simulink model "Copy_of_Scenario_MinimumExample_TwithoutTrafficLights"  (R2021a)
settings: Solver=VariableStepAuto  StartTime=0.0  StopTime=10.0  RelTol=1e-3
model workspace (MAT data in the model file):
  Kz_dif : Simulink.Parameter (value not decoded)
  Kz_il : Simulink.Parameter (value not decoded)
  Kz_ir : Simulink.Parameter (value not decoded)
  Kz_is : Simulink.Parameter (value not decoded)
  Kz_long : Simulink.Parameter (value not decoded)
  Kz_pre : Simulink.Parameter (value not decoded)
  L_dif : Simulink.Parameter (value not decoded)
  L_il : Simulink.Parameter (value not decoded)
  L_ir : Simulink.Parameter (value not decoded)
  L_is : Simulink.Parameter (value not decoded)
  L_long : Simulink.Parameter (value not decoded)
  L_pre : Simulink.Parameter (value not decoded)
  Lc : Simulink.Parameter (value not decoded)
  Rk : Simulink.Parameter (value not decoded)
  Tz_dif : Simulink.Parameter (value not decoded)
  Tz_il : Simulink.Parameter (value not decoded)
  Tz_ir : Simulink.Parameter (value not decoded)
  Tz_is : Simulink.Parameter (value not decoded)
  Tz_long : Simulink.Parameter (value not decoded)
  Tz_pre : Simulink.Parameter (value not decoded)
  ds : Simulink.Parameter (value not decoded)
  dt : Simulink.Parameter (value not decoded)
  v : Simulink.Parameter (value not decoded)
symbols that are objects in the model workspace (value not decoded): Kz_dif, Kz_il, Kz_ir, Kz_is, Kz_long, Kz_pre, Rk, Tz_dif, Tz_il, Tz_ir, Tz_is, Tz_long, Tz_pre
undefined symbols (not defined in the file): green_duration_l
libraries: StreetLanesLibrary x72, EdgesLibrary x58, SourcesAndSinksLibrary x12, simulink x12, LightsLibrary x2
(part 2 of 2)

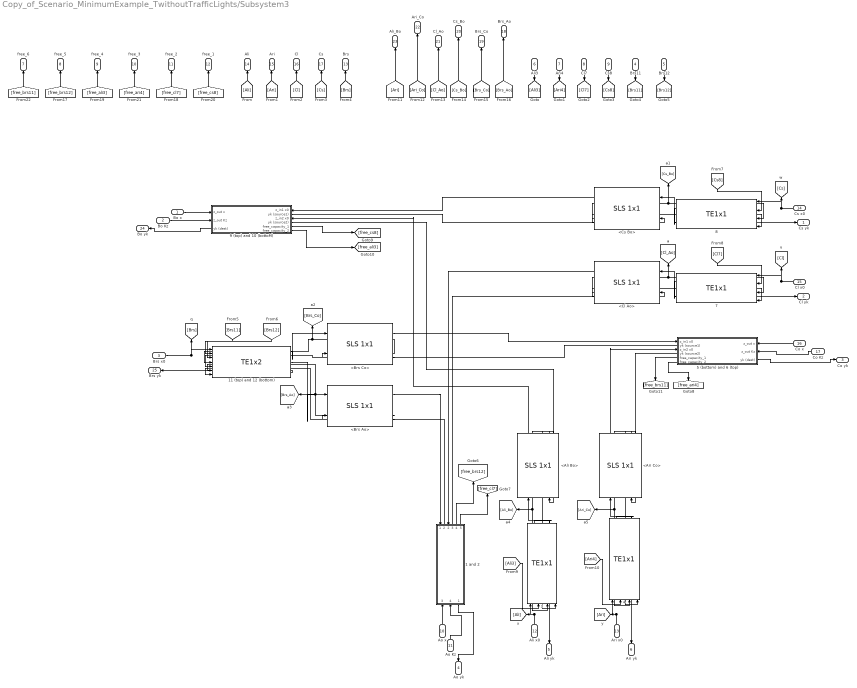
== system Copy_of_Scenario_MinimumExample_TwithoutTrafficLights/Subsystem3 ==
  Bo x : Inport
  Bo Kz : Inport  Port=2
  Brs x0 : Inport  Port=3
  Brs11 : Inport  Port=4
  Brs12 : Inport  Port=5
  Ali3 : Inport  Port=6
  Ari4 : Inport  Port=7
  Cl7 : Inport  Port=8
  Cs8 : Inport  Port=9
  Ao x : Inport  Port=10
  Ao Kz : Inport  Port=11
  Ali x0 : Inport  Port=12
  Ari x0 : Inport  Port=13
  Cs x0 : Inport  Port=14
  Cl x0 : Inport  Port=15
  Co x : Inport  Port=16
  Co Kz : Inport  Port=17
  1 and 2 : Subsystem  AncestorBlock=EdgesLibrary/SE2x1  mask{Rk1=Rk, Rk2=Rk}
      mask prompts: Rk1 "Rk (input 1)"; Rk2 "Rk (input 2)"
      settings: PortSchema="{\"entries\":[{\"content\":{\"sides\":[{\"content\":{\"connectorIds\":[\"In1\",\"Out2\",\"In2\",\"Out3\",\"Out4\",\"Out5\"]},\"type\":\"ConnectorPlacement.EquallySpacedRectSide\",\"uuid\":\"eb102e1f-8f68-4819-b192-9ed8ea7965cd\"},{\"content\":{\"connectorIds\":[\"In3\",\"In4\",\"Out1\"],\"side\":\"RIGHT\"},\"type\":\"ConnectorPlacement.EquallySpacedRectSide\",\"uuid\":\"0a8d41cc-2128-49e0-9ce9-20439c8bfca2\"},{\"content\":{\"connectorIds\":[],\"side\":\"TOP\"},\"type\":\"ConnectorPlacement.EquallySpacedRectSide\",\"uuid\":\"ce1e229b-7216-4f3c-b1ef-7720ca51f1c4\"}]},\"type\":\"ConnectorPlacement.EquallySpacedConnector\",\"uuid\":\"c8e8c67c-b38f-484f-95e7-011277152545\"}],\"packageUris\":[\"http://schema.mathworks.com/mf0/Connector/R2020b\"],\"version\":\"1.0\"}"
      mask Display:
      | image('$imagefile'); % Use "Edit Image" on toolstrip to change.
      | disp('Simple Edge 2x1\n\n\n');
      | Rk1 = get_param(gcb,'Rk1');
      | Rk2 = get_param(gcb, 'Rk2');
      | disp(['Rk1 = ', Rk1, ' | Rk2 =  ', Rk2])
  11 (top) and 12 (bottom) : EdgesLibrary/TE1x2  Rk1=0.5*Rk  Rk2=0.5*Rk
  {3..4,7..8} (4 alike) : EdgesLibrary/TE1x1  Rk=Rk
  5 (bottom) and 6 (top) : Subsystem  AncestorBlock=EdgesLibrary/SE2x1  mask{Rk1=Rk, Rk2=Rk}
      mask prompts: Rk1 "Rk (input 1)"; Rk2 "Rk (input 2)"
      settings: PortSchema="{\"entries\":[{\"content\":{\"sides\":[{\"content\":{\"connectorIds\":[\"In1\",\"Out2\",\"In2\",\"Out3\",\"Out4\",\"Out5\"]},\"type\":\"ConnectorPlacement.EquallySpacedRectSide\",\"uuid\":\"eb102e1f-8f68-4819-b192-9ed8ea7965cd\"},{\"content\":{\"connectorIds\":[\"In3\",\"In4\",\"Out1\"],\"side\":\"RIGHT\"},\"type\":\"ConnectorPlacement.EquallySpacedRectSide\",\"uuid\":\"0a8d41cc-2128-49e0-9ce9-20439c8bfca2\"},{\"content\":{\"connectorIds\":[],\"side\":\"TOP\"},\"type\":\"ConnectorPlacement.EquallySpacedRectSide\",\"uuid\":\"ce1e229b-7216-4f3c-b1ef-7720ca51f1c4\"}]},\"type\":\"ConnectorPlacement.EquallySpacedConnector\",\"uuid\":\"c8e8c67c-b38f-484f-95e7-011277152545\"}],\"packageUris\":[\"http://schema.mathworks.com/mf0/Connector/R2020b\"],\"version\":\"1.0\"}"
      mask Display:
      | image('$imagefile'); % Use "Edit Image" on toolstrip to change.
      | disp('Simple Edge 2x1\n\n\n');
      | Rk1 = get_param(gcb,'Rk1');
      | Rk2 = get_param(gcb, 'Rk2');
      | disp(['Rk1 = ', Rk1, ' | Rk2 =  ', Rk2])
  9 (top) and 10 (bottoM) : Subsystem  AncestorBlock=EdgesLibrary/SE2x1  mask{Rk1=Rk, Rk2=Rk}
      mask prompts: Rk1 "Rk (input 1)"; Rk2 "Rk (input 2)"
      settings: PortSchema="{\"entries\":[{\"content\":{\"sides\":[{\"content\":{\"connectorIds\":[\"In1\",\"Out2\",\"In2\",\"Out3\",\"Out4\",\"Out5\"]},\"type\":\"ConnectorPlacement.EquallySpacedRectSide\",\"uuid\":\"eb102e1f-8f68-4819-b192-9ed8ea7965cd\"},{\"content\":{\"connectorIds\":[\"In3\",\"In4\",\"Out1\"],\"side\":\"RIGHT\"},\"type\":\"ConnectorPlacement.EquallySpacedRectSide\",\"uuid\":\"0a8d41cc-2128-49e0-9ce9-20439c8bfca2\"},{\"content\":{\"connectorIds\":[],\"side\":\"TOP\"},\"type\":\"ConnectorPlacement.EquallySpacedRectSide\",\"uuid\":\"ce1e229b-7216-4f3c-b1ef-7720ca51f1c4\"}]},\"type\":\"ConnectorPlacement.EquallySpacedConnector\",\"uuid\":\"c8e8c67c-b38f-484f-95e7-011277152545\"}],\"packageUris\":[\"http://schema.mathworks.com/mf0/Connector/R2020b\"],\"version\":\"1.0\"}"
      mask Display:
      | image('$imagefile'); % Use "Edit Image" on toolstrip to change.
      | disp('Simple Edge 2x1\n\n\n');
      | Rk1 = get_param(gcb,'Rk1');
      | Rk2 = get_param(gcb, 'Rk2');
      | disp(['Rk1 = ', Rk1, ' | Rk2 =  ', Rk2])
  <Ali Bo> : StreetLanesLibrary/SLS 1x1  Kz=Kz_left  Tz=Tz_left
  <Ari Co> : StreetLanesLibrary/SLS 1x1  Kz=Kz_right  Tz=Tz_right
  <Brs Ao> : StreetLanesLibrary/SLS 1x1  Kz=Kz_right  Tz=Tz_right
  <Brs Co> : StreetLanesLibrary/SLS 1x1  Kz=Kz_straight  Tz=Tz_straight
  <Cl Ao> : StreetLanesLibrary/SLS 1x1  Kz=Kz_left  Tz=Tz_left
  <Cs Bo> : StreetLanesLibrary/SLS 1x1  Kz=Kz_straight  Tz=Tz_straight
  Cs yk : Outport
  Cl yk : Outport  Port=2
  Co yk : Outport  Port=3
  Ao yk : Outport  Port=4
  Ali yk : Outport  Port=5
  Ari yk : Outport  Port=6
  free_6 : Outport  Port=7
  free_5 : Outport  Port=8
  free_4 : Outport  Port=9
  free_3 : Outport  Port=10
  free_2 : Outport  Port=11
  free_1 : Outport  Port=12
  Brs : Outport  Port=13
  Ali : Outport  Port=14
  Ari : Outport  Port=15
  Cl : Outport  Port=16
  Cs : Outport  Port=17
  Brs_Ao : Outport  Port=18
  Brs_Co : Outport  Port=19
  Cs_Bo : Outport  Port=20
  Cl_Ao : Outport  Port=21
  Ari_Co : Outport  Port=22
  Ali_Bo : Outport  Port=23
  Bo yk : Outport  Port=24
  Brs yk : Outport  Port=25
  wires:
  11 (top) and 12 (bottom)/2 -> <Brs Ao>/1
  11 (top) and 12 (bottom)/3 -> Brs yk/1
  3/2 -> Ali yk/1
  3/1 -> <Ali Bo>/1
  Ari x0/1 -> [Ari], 4/1
  <Cs Bo>/2 -> 9 (top) and 10 (bottoM)/1(z_in1 x0)
  <Cs Bo>/8 -> 8/4
  <Cl Ao>/8 -> 7/4
  Co x/1 -> 5 (bottom) and 6 (top)/3(z_out x)
  5 (bottom) and 6 (top)/1(yk (dest)) -> Co yk/1
  5 (bottom) and 6 (top)/3(yk (source2)) -> <Ari Co>/2
  <Ari Co>/8 -> 4/4
  <Ali Bo>/8 -> 3/4
  Ao x/1 -> 1 and 2/3(z_out x)
  Brs x0/1 -> 11 (top) and 12 (bottom)/1, [Brs]
  <Brs Co>/2 -> 5 (bottom) and 6 (top)/1(z_in1 x0)
  <Cl Ao>/7 -> [Cl_Ao], 7/3
  <Cl Ao>/2 -> 1 and 2/2(z_in2 x0)
  9 (top) and 10 (bottoM)/2(yk (source1)) -> <Cs Bo>/2
  <Ari Co>/2 -> 5 (bottom) and 6 (top)/2(z_in2 x0)
  7/1 -> <Cl Ao>/1
  Cl x0/1 -> [Cl], 7/1
  4/1 -> <Ari Co>/1
  <Ari Co>/7 -> 4/3, [Ari_Co]
  <Brs Ao>/2 -> 1 and 2/1(z_in1 x0)
  Ao Kz/1 -> 1 and 2/4(z_out Kz)
  <Brs Ao>/7 -> [Brs_Ao], 11 (top) and 12 (bottom)/6
  <Brs Ao>/8 -> 11 (top) and 12 (bottom)/7
  Co Kz/1 -> 5 (bottom) and 6 (top)/4(z_out Kz)
  8/2 -> Cs yk/1
  Bo Kz/1 -> 9 (top) and 10 (bottoM)/4(z_out Kz)
  1 and 2/3(yk (source2)) -> <Cl Ao>/2
  <Brs Co>/8 -> 11 (top) and 12 (bottom)/5
  [Brs12] -> 11 (top) and 12 (bottom)/3
  9 (top) and 10 (bottoM)/3(yk (source2)) -> <Ali Bo>/2
  <Ali Bo>/7 -> 3/3, [Ali_Bo]
  1 and 2/2(yk (source1)) -> <Brs Ao>/2
  Ali x0/1 -> [Ali], 3/1
  <Brs Co>/7 -> 11 (top) and 12 (bottom)/4, [Brs_Co]
  1 and 2/1(yk (dest)) -> Ao yk/1
  <Ali Bo>/2 -> 9 (top) and 10 (bottoM)/2(z_in2 x0)
  [Ari4] -> 4/2
  5 (bottom) and 6 (top)/2(yk (source1)) -> <Brs Co>/2
  8/1 -> <Cs Bo>/1
  4/2 -> Ari yk/1
  <Cs Bo>/7 -> 8/3, [Cs_Bo]
  Cs x0/1 -> [Cs], 8/1
  [Ali3] -> 3/2
  [Brs11] -> 11 (top) and 12 (bottom)/2
  11 (top) and 12 (bottom)/1 -> <Brs Co>/1
  Bo x/1 -> 9 (top) and 10 (bottoM)/3(z_out x)
  [Cl7] -> 7/2
  9 (top) and 10 (bottoM)/1(yk (dest)) -> Bo yk/1
  7/2 -> Cl yk/1
  [Cs8] -> 8/2
  [Ari] -> Ali_Bo/1
  [Ari_Co] -> Ari_Co/1
  [Cl_Ao] -> Cl_Ao/1
  [Cs_Bo] -> Cs_Bo/1
  [Brs_Co] -> Brs_Co/1
  [Brs_Ao] -> Brs_Ao/1
  [Ali] -> Ali/1
  [Ari] -> Ari/1
  [Cl] -> Cl/1
  [Cs] -> Cs/1
  [Brs] -> Brs/1
  Ali3/1 -> [Ali3]
  Ari4/1 -> [Ari4]
  Cl7/1 -> [Cl7]
  Cs8/1 -> [Cs8]
  Brs11/1 -> [Brs11]
  Brs12/1 -> [Brs12]
  1 and 2/4(free_capacity_1) -> [free_brs12]
  1 and 2/5(free_capacity_2) -> [free_cl7]
  9 (top) and 10 (bottoM)/4(free_capacity_1) -> [free_cs8]
  9 (top) and 10 (bottoM)/5(free_capacity_2) -> [free_ali3]
  5 (bottom) and 6 (top)/5(free_capacity_2) -> [free_ari4]
  5 (bottom) and 6 (top)/4(free_capacity_1) -> [free_brs11]
  [free_cs8] -> free_1/1
  [free_cl7] -> free_2/1
  [free_ari4] -> free_3/1
  [free_ali3] -> free_4/1
  [free_brs12] -> free_5/1
  [free_brs11] -> free_6/1

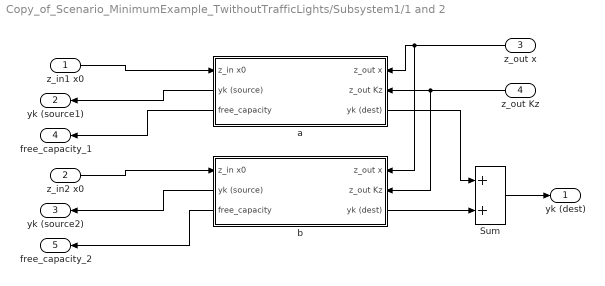
== system Copy_of_Scenario_MinimumExample_TwithoutTrafficLights/Subsystem1/1 and 2 ==
  z_in1 x0 : Inport
  z_in2 x0 : Inport  Port=2
  z_out x : Inport  Port=3
  z_out Kz : Inport  Port=4
  Sum : Sum
  a : Subsystem  AncestorBlock=EdgesLibrary/SE1x1  mask{Rk=Rk1}
      mask prompts: Rk "Rk (fixed flowrate, used when the flow is enabled)"
      mask help: This block serves to establish a flow between two Street Lane Segments. To archieve this, it connects one source-cell [z_in] to one destination-cell [z_out], and prompts a flow of cars with the rate Rk (Parameter) if and only if there are still cars at the end of [z_out] avaiable and if the capacity of [z_out] is not yet surpassed, i.e. (z_in x0 > 0 AND z_out Kz > z_out x), otherwise the flow is reduced to 0.
      settings: PortSchema="{\"entries\":[{\"content\":{\"sides\":[{\"content\":{\"connectorIds\":[\"In1\",\"Out2\",\"Out3\"]},\"type\":\"ConnectorPlacement.EquallySpacedRectSide\",\"uuid\":\"f9c1cf46-46ac-4011-8499-7a2e74fc4a3a\"},{\"content\":{\"connectorIds\":[\"In2\",\"In3\",\"Out1\"],\"side\":\"RIGHT\"},\"type\":\"ConnectorPlacement.EquallySpacedRectSide\",\"uuid\":\"f685a77a-a8b9-4a29-8679-dc3cbf3c2b7f\"},{\"content\":{\"connectorIds\":[],\"side\":\"TOP\"},\"type\":\"ConnectorPlacement.EquallySpacedRectSide\",\"uuid\":\"af8d715a-ddb3-4f5e-8163-596be4e65ef7\"}]},\"type\":\"ConnectorPlacement.EquallySpacedConnector\",\"uuid\":\"ace495d2-b7cd-4153-a555-4989f077c969\"}],\"packageUris\":[\"http://schema.mathworks.com/mf0/Connector/R2020b\"],\"version\":\"1.0\"}"
      mask Display:
      | image('$imagefile'); % Use "Edit Image" on toolstrip to change.
      | % image('$imagefile');
      | disp('Simple Edge 1x1 \n\n');
      | disp(['Rk = ', get_param(gcb,'Rk')])
  b : Subsystem  AncestorBlock=EdgesLibrary/SE1x1  mask{Rk=Rk2}
      mask prompts: Rk "Rk (fixed flowrate, used when the flow is enabled)"
      mask help: This block serves to establish a flow between two Street Lane Segments. To archieve this, it connects one source-cell [z_in] to one destination-cell [z_out], and prompts a flow of cars with the rate Rk (Parameter) if and only if there are still cars at the end of [z_out] avaiable and if the capacity of [z_out] is not yet surpassed, i.e. (z_in x0 > 0 AND z_out Kz > z_out x), otherwise the flow is reduced to 0.
      settings: PortSchema="{\"entries\":[{\"content\":{\"sides\":[{\"content\":{\"connectorIds\":[\"In1\",\"Out2\",\"Out3\"]},\"type\":\"ConnectorPlacement.EquallySpacedRectSide\",\"uuid\":\"f9c1cf46-46ac-4011-8499-7a2e74fc4a3a\"},{\"content\":{\"connectorIds\":[\"In2\",\"In3\",\"Out1\"],\"side\":\"RIGHT\"},\"type\":\"ConnectorPlacement.EquallySpacedRectSide\",\"uuid\":\"f685a77a-a8b9-4a29-8679-dc3cbf3c2b7f\"},{\"content\":{\"connectorIds\":[],\"side\":\"TOP\"},\"type\":\"ConnectorPlacement.EquallySpacedRectSide\",\"uuid\":\"af8d715a-ddb3-4f5e-8163-596be4e65ef7\"}]},\"type\":\"ConnectorPlacement.EquallySpacedConnector\",\"uuid\":\"ace495d2-b7cd-4153-a555-4989f077c969\"}],\"packageUris\":[\"http://schema.mathworks.com/mf0/Connector/R2020b\"],\"version\":\"1.0\"}"
      mask Display:
      | image('$imagefile'); % Use "Edit Image" on toolstrip to change.
      | % image('$imagefile');
      | disp('Simple Edge 1x1 \n\n');
      | disp(['Rk = ', get_param(gcb,'Rk')])
  yk (dest) : Outport
  yk (source1) : Outport  Port=2
  yk (source2) : Outport  Port=3
  free_capacity_1 : Outport  Port=4
  free_capacity_2 : Outport  Port=5
  wires:
  z_out Kz/1 -> b/3(z_out Kz), a/3(z_out Kz)
  Sum/1 -> yk (dest)/1
  z_out x/1 -> b/2(z_out x), a/2(z_out x)
  b/1(yk (dest)) -> Sum/2
  z_in1 x0/1 -> a/1(z_in x0)
  a/1(yk (dest)) -> Sum/1
  z_in2 x0/1 -> b/1(z_in x0)
  b/2(yk (source)) -> yk (source2)/1
  a/2(yk (source)) -> yk (source1)/1
  a/3(free_capacity) -> free_capacity_1/1
  b/3(free_capacity) -> free_capacity_2/1

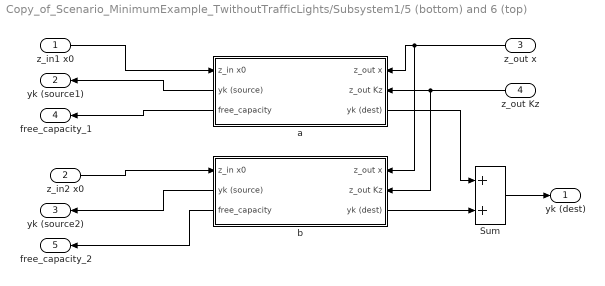
== system Copy_of_Scenario_MinimumExample_TwithoutTrafficLights/Subsystem1/5 (bottom) and 6 (top) ==
  z_in1 x0 : Inport
  z_in2 x0 : Inport  Port=2
  z_out x : Inport  Port=3
  z_out Kz : Inport  Port=4
  Sum : Sum
  a : Subsystem  AncestorBlock=EdgesLibrary/SE1x1  mask{Rk=Rk1}
      mask prompts: Rk "Rk (fixed flowrate, used when the flow is enabled)"
      mask help: This block serves to establish a flow between two Street Lane Segments. To archieve this, it connects one source-cell [z_in] to one destination-cell [z_out], and prompts a flow of cars with the rate Rk (Parameter) if and only if there are still cars at the end of [z_out] avaiable and if the capacity of [z_out] is not yet surpassed, i.e. (z_in x0 > 0 AND z_out Kz > z_out x), otherwise the flow is reduced to 0.
      settings: PortSchema="{\"entries\":[{\"content\":{\"sides\":[{\"content\":{\"connectorIds\":[\"In1\",\"Out2\",\"Out3\"]},\"type\":\"ConnectorPlacement.EquallySpacedRectSide\",\"uuid\":\"f9c1cf46-46ac-4011-8499-7a2e74fc4a3a\"},{\"content\":{\"connectorIds\":[\"In2\",\"In3\",\"Out1\"],\"side\":\"RIGHT\"},\"type\":\"ConnectorPlacement.EquallySpacedRectSide\",\"uuid\":\"f685a77a-a8b9-4a29-8679-dc3cbf3c2b7f\"},{\"content\":{\"connectorIds\":[],\"side\":\"TOP\"},\"type\":\"ConnectorPlacement.EquallySpacedRectSide\",\"uuid\":\"af8d715a-ddb3-4f5e-8163-596be4e65ef7\"}]},\"type\":\"ConnectorPlacement.EquallySpacedConnector\",\"uuid\":\"ace495d2-b7cd-4153-a555-4989f077c969\"}],\"packageUris\":[\"http://schema.mathworks.com/mf0/Connector/R2020b\"],\"version\":\"1.0\"}"
      mask Display:
      | image('$imagefile'); % Use "Edit Image" on toolstrip to change.
      | % image('$imagefile');
      | disp('Simple Edge 1x1 \n\n');
      | disp(['Rk = ', get_param(gcb,'Rk')])
  b : Subsystem  AncestorBlock=EdgesLibrary/SE1x1  mask{Rk=Rk2}
      mask prompts: Rk "Rk (fixed flowrate, used when the flow is enabled)"
      mask help: This block serves to establish a flow between two Street Lane Segments. To archieve this, it connects one source-cell [z_in] to one destination-cell [z_out], and prompts a flow of cars with the rate Rk (Parameter) if and only if there are still cars at the end of [z_out] avaiable and if the capacity of [z_out] is not yet surpassed, i.e. (z_in x0 > 0 AND z_out Kz > z_out x), otherwise the flow is reduced to 0.
      settings: PortSchema="{\"entries\":[{\"content\":{\"sides\":[{\"content\":{\"connectorIds\":[\"In1\",\"Out2\",\"Out3\"]},\"type\":\"ConnectorPlacement.EquallySpacedRectSide\",\"uuid\":\"f9c1cf46-46ac-4011-8499-7a2e74fc4a3a\"},{\"content\":{\"connectorIds\":[\"In2\",\"In3\",\"Out1\"],\"side\":\"RIGHT\"},\"type\":\"ConnectorPlacement.EquallySpacedRectSide\",\"uuid\":\"f685a77a-a8b9-4a29-8679-dc3cbf3c2b7f\"},{\"content\":{\"connectorIds\":[],\"side\":\"TOP\"},\"type\":\"ConnectorPlacement.EquallySpacedRectSide\",\"uuid\":\"af8d715a-ddb3-4f5e-8163-596be4e65ef7\"}]},\"type\":\"ConnectorPlacement.EquallySpacedConnector\",\"uuid\":\"ace495d2-b7cd-4153-a555-4989f077c969\"}],\"packageUris\":[\"http://schema.mathworks.com/mf0/Connector/R2020b\"],\"version\":\"1.0\"}"
      mask Display:
      | image('$imagefile'); % Use "Edit Image" on toolstrip to change.
      | % image('$imagefile');
      | disp('Simple Edge 1x1 \n\n');
      | disp(['Rk = ', get_param(gcb,'Rk')])
  yk (dest) : Outport
  yk (source1) : Outport  Port=2
  yk (source2) : Outport  Port=3
  free_capacity_1 : Outport  Port=4
  free_capacity_2 : Outport  Port=5
  wires:
  z_out Kz/1 -> b/3(z_out Kz), a/3(z_out Kz)
  Sum/1 -> yk (dest)/1
  z_out x/1 -> b/2(z_out x), a/2(z_out x)
  b/1(yk (dest)) -> Sum/2
  z_in1 x0/1 -> a/1(z_in x0)
  a/1(yk (dest)) -> Sum/1
  z_in2 x0/1 -> b/1(z_in x0)
  b/2(yk (source)) -> yk (source2)/1
  a/2(yk (source)) -> yk (source1)/1
  a/3(free_capacity) -> free_capacity_1/1
  b/3(free_capacity) -> free_capacity_2/1

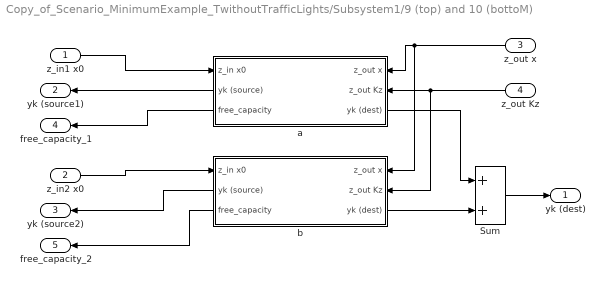
== system Copy_of_Scenario_MinimumExample_TwithoutTrafficLights/Subsystem1/9 (top) and 10 (bottoM) ==
  z_in1 x0 : Inport
  z_in2 x0 : Inport  Port=2
  z_out x : Inport  Port=3
  z_out Kz : Inport  Port=4
  Sum : Sum
  a : Subsystem  AncestorBlock=EdgesLibrary/SE1x1  mask{Rk=Rk1}
      mask prompts: Rk "Rk (fixed flowrate, used when the flow is enabled)"
      mask help: This block serves to establish a flow between two Street Lane Segments. To archieve this, it connects one source-cell [z_in] to one destination-cell [z_out], and prompts a flow of cars with the rate Rk (Parameter) if and only if there are still cars at the end of [z_out] avaiable and if the capacity of [z_out] is not yet surpassed, i.e. (z_in x0 > 0 AND z_out Kz > z_out x), otherwise the flow is reduced to 0.
      settings: PortSchema="{\"entries\":[{\"content\":{\"sides\":[{\"content\":{\"connectorIds\":[\"In1\",\"Out2\",\"Out3\"]},\"type\":\"ConnectorPlacement.EquallySpacedRectSide\",\"uuid\":\"f9c1cf46-46ac-4011-8499-7a2e74fc4a3a\"},{\"content\":{\"connectorIds\":[\"In2\",\"In3\",\"Out1\"],\"side\":\"RIGHT\"},\"type\":\"ConnectorPlacement.EquallySpacedRectSide\",\"uuid\":\"f685a77a-a8b9-4a29-8679-dc3cbf3c2b7f\"},{\"content\":{\"connectorIds\":[],\"side\":\"TOP\"},\"type\":\"ConnectorPlacement.EquallySpacedRectSide\",\"uuid\":\"af8d715a-ddb3-4f5e-8163-596be4e65ef7\"}]},\"type\":\"ConnectorPlacement.EquallySpacedConnector\",\"uuid\":\"ace495d2-b7cd-4153-a555-4989f077c969\"}],\"packageUris\":[\"http://schema.mathworks.com/mf0/Connector/R2020b\"],\"version\":\"1.0\"}"
      mask Display:
      | image('$imagefile'); % Use "Edit Image" on toolstrip to change.
      | % image('$imagefile');
      | disp('Simple Edge 1x1 \n\n');
      | disp(['Rk = ', get_param(gcb,'Rk')])
  b : Subsystem  AncestorBlock=EdgesLibrary/SE1x1  mask{Rk=Rk2}
      mask prompts: Rk "Rk (fixed flowrate, used when the flow is enabled)"
      mask help: This block serves to establish a flow between two Street Lane Segments. To archieve this, it connects one source-cell [z_in] to one destination-cell [z_out], and prompts a flow of cars with the rate Rk (Parameter) if and only if there are still cars at the end of [z_out] avaiable and if the capacity of [z_out] is not yet surpassed, i.e. (z_in x0 > 0 AND z_out Kz > z_out x), otherwise the flow is reduced to 0.
      settings: PortSchema="{\"entries\":[{\"content\":{\"sides\":[{\"content\":{\"connectorIds\":[\"In1\",\"Out2\",\"Out3\"]},\"type\":\"ConnectorPlacement.EquallySpacedRectSide\",\"uuid\":\"f9c1cf46-46ac-4011-8499-7a2e74fc4a3a\"},{\"content\":{\"connectorIds\":[\"In2\",\"In3\",\"Out1\"],\"side\":\"RIGHT\"},\"type\":\"ConnectorPlacement.EquallySpacedRectSide\",\"uuid\":\"f685a77a-a8b9-4a29-8679-dc3cbf3c2b7f\"},{\"content\":{\"connectorIds\":[],\"side\":\"TOP\"},\"type\":\"ConnectorPlacement.EquallySpacedRectSide\",\"uuid\":\"af8d715a-ddb3-4f5e-8163-596be4e65ef7\"}]},\"type\":\"ConnectorPlacement.EquallySpacedConnector\",\"uuid\":\"ace495d2-b7cd-4153-a555-4989f077c969\"}],\"packageUris\":[\"http://schema.mathworks.com/mf0/Connector/R2020b\"],\"version\":\"1.0\"}"
      mask Display:
      | image('$imagefile'); % Use "Edit Image" on toolstrip to change.
      | % image('$imagefile');
      | disp('Simple Edge 1x1 \n\n');
      | disp(['Rk = ', get_param(gcb,'Rk')])
  yk (dest) : Outport
  yk (source1) : Outport  Port=2
  yk (source2) : Outport  Port=3
  free_capacity_1 : Outport  Port=4
  free_capacity_2 : Outport  Port=5
  wires:
  z_out Kz/1 -> b/3(z_out Kz), a/3(z_out Kz)
  Sum/1 -> yk (dest)/1
  z_out x/1 -> b/2(z_out x), a/2(z_out x)
  b/1(yk (dest)) -> Sum/2
  z_in1 x0/1 -> a/1(z_in x0)
  a/1(yk (dest)) -> Sum/1
  z_in2 x0/1 -> b/1(z_in x0)
  b/2(yk (source)) -> yk (source2)/1
  a/2(yk (source)) -> yk (source1)/1
  a/3(free_capacity) -> free_capacity_1/1
  b/3(free_capacity) -> free_capacity_2/1

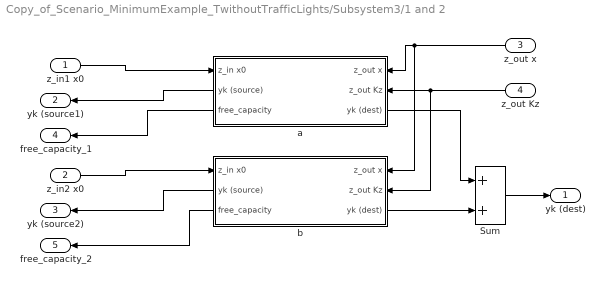
== system Copy_of_Scenario_MinimumExample_TwithoutTrafficLights/Subsystem3/1 and 2 ==
  z_in1 x0 : Inport
  z_in2 x0 : Inport  Port=2
  z_out x : Inport  Port=3
  z_out Kz : Inport  Port=4
  Sum : Sum
  a : Subsystem  AncestorBlock=EdgesLibrary/SE1x1  mask{Rk=Rk1}
      mask prompts: Rk "Rk (fixed flowrate, used when the flow is enabled)"
      mask help: This block serves to establish a flow between two Street Lane Segments. To archieve this, it connects one source-cell [z_in] to one destination-cell [z_out], and prompts a flow of cars with the rate Rk (Parameter) if and only if there are still cars at the end of [z_out] avaiable and if the capacity of [z_out] is not yet surpassed, i.e. (z_in x0 > 0 AND z_out Kz > z_out x), otherwise the flow is reduced to 0.
      settings: PortSchema="{\"entries\":[{\"content\":{\"sides\":[{\"content\":{\"connectorIds\":[\"In1\",\"Out2\",\"Out3\"]},\"type\":\"ConnectorPlacement.EquallySpacedRectSide\",\"uuid\":\"f9c1cf46-46ac-4011-8499-7a2e74fc4a3a\"},{\"content\":{\"connectorIds\":[\"In2\",\"In3\",\"Out1\"],\"side\":\"RIGHT\"},\"type\":\"ConnectorPlacement.EquallySpacedRectSide\",\"uuid\":\"f685a77a-a8b9-4a29-8679-dc3cbf3c2b7f\"},{\"content\":{\"connectorIds\":[],\"side\":\"TOP\"},\"type\":\"ConnectorPlacement.EquallySpacedRectSide\",\"uuid\":\"af8d715a-ddb3-4f5e-8163-596be4e65ef7\"}]},\"type\":\"ConnectorPlacement.EquallySpacedConnector\",\"uuid\":\"ace495d2-b7cd-4153-a555-4989f077c969\"}],\"packageUris\":[\"http://schema.mathworks.com/mf0/Connector/R2020b\"],\"version\":\"1.0\"}"
      mask Display:
      | image('$imagefile'); % Use "Edit Image" on toolstrip to change.
      | % image('$imagefile');
      | disp('Simple Edge 1x1 \n\n');
      | disp(['Rk = ', get_param(gcb,'Rk')])
  b : Subsystem  AncestorBlock=EdgesLibrary/SE1x1  mask{Rk=Rk2}
      mask prompts: Rk "Rk (fixed flowrate, used when the flow is enabled)"
      mask help: This block serves to establish a flow between two Street Lane Segments. To archieve this, it connects one source-cell [z_in] to one destination-cell [z_out], and prompts a flow of cars with the rate Rk (Parameter) if and only if there are still cars at the end of [z_out] avaiable and if the capacity of [z_out] is not yet surpassed, i.e. (z_in x0 > 0 AND z_out Kz > z_out x), otherwise the flow is reduced to 0.
      settings: PortSchema="{\"entries\":[{\"content\":{\"sides\":[{\"content\":{\"connectorIds\":[\"In1\",\"Out2\",\"Out3\"]},\"type\":\"ConnectorPlacement.EquallySpacedRectSide\",\"uuid\":\"f9c1cf46-46ac-4011-8499-7a2e74fc4a3a\"},{\"content\":{\"connectorIds\":[\"In2\",\"In3\",\"Out1\"],\"side\":\"RIGHT\"},\"type\":\"ConnectorPlacement.EquallySpacedRectSide\",\"uuid\":\"f685a77a-a8b9-4a29-8679-dc3cbf3c2b7f\"},{\"content\":{\"connectorIds\":[],\"side\":\"TOP\"},\"type\":\"ConnectorPlacement.EquallySpacedRectSide\",\"uuid\":\"af8d715a-ddb3-4f5e-8163-596be4e65ef7\"}]},\"type\":\"ConnectorPlacement.EquallySpacedConnector\",\"uuid\":\"ace495d2-b7cd-4153-a555-4989f077c969\"}],\"packageUris\":[\"http://schema.mathworks.com/mf0/Connector/R2020b\"],\"version\":\"1.0\"}"
      mask Display:
      | image('$imagefile'); % Use "Edit Image" on toolstrip to change.
      | % image('$imagefile');
      | disp('Simple Edge 1x1 \n\n');
      | disp(['Rk = ', get_param(gcb,'Rk')])
  yk (dest) : Outport
  yk (source1) : Outport  Port=2
  yk (source2) : Outport  Port=3
  free_capacity_1 : Outport  Port=4
  free_capacity_2 : Outport  Port=5
  wires:
  z_out Kz/1 -> b/3(z_out Kz), a/3(z_out Kz)
  Sum/1 -> yk (dest)/1
  z_out x/1 -> b/2(z_out x), a/2(z_out x)
  b/1(yk (dest)) -> Sum/2
  z_in1 x0/1 -> a/1(z_in x0)
  a/1(yk (dest)) -> Sum/1
  z_in2 x0/1 -> b/1(z_in x0)
  b/2(yk (source)) -> yk (source2)/1
  a/2(yk (source)) -> yk (source1)/1
  a/3(free_capacity) -> free_capacity_1/1
  b/3(free_capacity) -> free_capacity_2/1

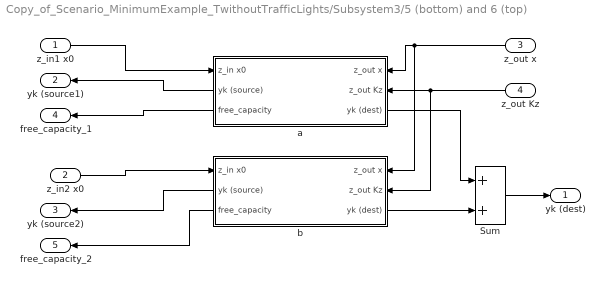
== system Copy_of_Scenario_MinimumExample_TwithoutTrafficLights/Subsystem3/5 (bottom) and 6 (top) ==
  z_in1 x0 : Inport
  z_in2 x0 : Inport  Port=2
  z_out x : Inport  Port=3
  z_out Kz : Inport  Port=4
  Sum : Sum
  a : Subsystem  AncestorBlock=EdgesLibrary/SE1x1  mask{Rk=Rk1}
      mask prompts: Rk "Rk (fixed flowrate, used when the flow is enabled)"
      mask help: This block serves to establish a flow between two Street Lane Segments. To archieve this, it connects one source-cell [z_in] to one destination-cell [z_out], and prompts a flow of cars with the rate Rk (Parameter) if and only if there are still cars at the end of [z_out] avaiable and if the capacity of [z_out] is not yet surpassed, i.e. (z_in x0 > 0 AND z_out Kz > z_out x), otherwise the flow is reduced to 0.
      settings: PortSchema="{\"entries\":[{\"content\":{\"sides\":[{\"content\":{\"connectorIds\":[\"In1\",\"Out2\",\"Out3\"]},\"type\":\"ConnectorPlacement.EquallySpacedRectSide\",\"uuid\":\"f9c1cf46-46ac-4011-8499-7a2e74fc4a3a\"},{\"content\":{\"connectorIds\":[\"In2\",\"In3\",\"Out1\"],\"side\":\"RIGHT\"},\"type\":\"ConnectorPlacement.EquallySpacedRectSide\",\"uuid\":\"f685a77a-a8b9-4a29-8679-dc3cbf3c2b7f\"},{\"content\":{\"connectorIds\":[],\"side\":\"TOP\"},\"type\":\"ConnectorPlacement.EquallySpacedRectSide\",\"uuid\":\"af8d715a-ddb3-4f5e-8163-596be4e65ef7\"}]},\"type\":\"ConnectorPlacement.EquallySpacedConnector\",\"uuid\":\"ace495d2-b7cd-4153-a555-4989f077c969\"}],\"packageUris\":[\"http://schema.mathworks.com/mf0/Connector/R2020b\"],\"version\":\"1.0\"}"
      mask Display:
      | image('$imagefile'); % Use "Edit Image" on toolstrip to change.
      | % image('$imagefile');
      | disp('Simple Edge 1x1 \n\n');
      | disp(['Rk = ', get_param(gcb,'Rk')])
  b : Subsystem  AncestorBlock=EdgesLibrary/SE1x1  mask{Rk=Rk2}
      mask prompts: Rk "Rk (fixed flowrate, used when the flow is enabled)"
      mask help: This block serves to establish a flow between two Street Lane Segments. To archieve this, it connects one source-cell [z_in] to one destination-cell [z_out], and prompts a flow of cars with the rate Rk (Parameter) if and only if there are still cars at the end of [z_out] avaiable and if the capacity of [z_out] is not yet surpassed, i.e. (z_in x0 > 0 AND z_out Kz > z_out x), otherwise the flow is reduced to 0.
      settings: PortSchema="{\"entries\":[{\"content\":{\"sides\":[{\"content\":{\"connectorIds\":[\"In1\",\"Out2\",\"Out3\"]},\"type\":\"ConnectorPlacement.EquallySpacedRectSide\",\"uuid\":\"f9c1cf46-46ac-4011-8499-7a2e74fc4a3a\"},{\"content\":{\"connectorIds\":[\"In2\",\"In3\",\"Out1\"],\"side\":\"RIGHT\"},\"type\":\"ConnectorPlacement.EquallySpacedRectSide\",\"uuid\":\"f685a77a-a8b9-4a29-8679-dc3cbf3c2b7f\"},{\"content\":{\"connectorIds\":[],\"side\":\"TOP\"},\"type\":\"ConnectorPlacement.EquallySpacedRectSide\",\"uuid\":\"af8d715a-ddb3-4f5e-8163-596be4e65ef7\"}]},\"type\":\"ConnectorPlacement.EquallySpacedConnector\",\"uuid\":\"ace495d2-b7cd-4153-a555-4989f077c969\"}],\"packageUris\":[\"http://schema.mathworks.com/mf0/Connector/R2020b\"],\"version\":\"1.0\"}"
      mask Display:
      | image('$imagefile'); % Use "Edit Image" on toolstrip to change.
      | % image('$imagefile');
      | disp('Simple Edge 1x1 \n\n');
      | disp(['Rk = ', get_param(gcb,'Rk')])
  yk (dest) : Outport
  yk (source1) : Outport  Port=2
  yk (source2) : Outport  Port=3
  free_capacity_1 : Outport  Port=4
  free_capacity_2 : Outport  Port=5
  wires:
  z_out Kz/1 -> b/3(z_out Kz), a/3(z_out Kz)
  Sum/1 -> yk (dest)/1
  z_out x/1 -> b/2(z_out x), a/2(z_out x)
  b/1(yk (dest)) -> Sum/2
  z_in1 x0/1 -> a/1(z_in x0)
  a/1(yk (dest)) -> Sum/1
  z_in2 x0/1 -> b/1(z_in x0)
  b/2(yk (source)) -> yk (source2)/1
  a/2(yk (source)) -> yk (source1)/1
  a/3(free_capacity) -> free_capacity_1/1
  b/3(free_capacity) -> free_capacity_2/1

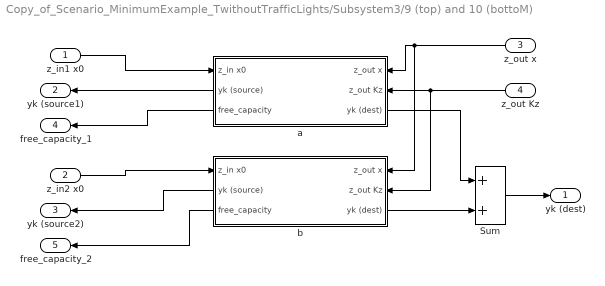
== system Copy_of_Scenario_MinimumExample_TwithoutTrafficLights/Subsystem3/9 (top) and 10 (bottoM) ==
  z_in1 x0 : Inport
  z_in2 x0 : Inport  Port=2
  z_out x : Inport  Port=3
  z_out Kz : Inport  Port=4
  Sum : Sum
  a : Subsystem  AncestorBlock=EdgesLibrary/SE1x1  mask{Rk=Rk1}
      mask prompts: Rk "Rk (fixed flowrate, used when the flow is enabled)"
      mask help: This block serves to establish a flow between two Street Lane Segments. To archieve this, it connects one source-cell [z_in] to one destination-cell [z_out], and prompts a flow of cars with the rate Rk (Parameter) if and only if there are still cars at the end of [z_out] avaiable and if the capacity of [z_out] is not yet surpassed, i.e. (z_in x0 > 0 AND z_out Kz > z_out x), otherwise the flow is reduced to 0.
      settings: PortSchema="{\"entries\":[{\"content\":{\"sides\":[{\"content\":{\"connectorIds\":[\"In1\",\"Out2\",\"Out3\"]},\"type\":\"ConnectorPlacement.EquallySpacedRectSide\",\"uuid\":\"f9c1cf46-46ac-4011-8499-7a2e74fc4a3a\"},{\"content\":{\"connectorIds\":[\"In2\",\"In3\",\"Out1\"],\"side\":\"RIGHT\"},\"type\":\"ConnectorPlacement.EquallySpacedRectSide\",\"uuid\":\"f685a77a-a8b9-4a29-8679-dc3cbf3c2b7f\"},{\"content\":{\"connectorIds\":[],\"side\":\"TOP\"},\"type\":\"ConnectorPlacement.EquallySpacedRectSide\",\"uuid\":\"af8d715a-ddb3-4f5e-8163-596be4e65ef7\"}]},\"type\":\"ConnectorPlacement.EquallySpacedConnector\",\"uuid\":\"ace495d2-b7cd-4153-a555-4989f077c969\"}],\"packageUris\":[\"http://schema.mathworks.com/mf0/Connector/R2020b\"],\"version\":\"1.0\"}"
      mask Display:
      | image('$imagefile'); % Use "Edit Image" on toolstrip to change.
      | % image('$imagefile');
      | disp('Simple Edge 1x1 \n\n');
      | disp(['Rk = ', get_param(gcb,'Rk')])
  b : Subsystem  AncestorBlock=EdgesLibrary/SE1x1  mask{Rk=Rk2}
      mask prompts: Rk "Rk (fixed flowrate, used when the flow is enabled)"
      mask help: This block serves to establish a flow between two Street Lane Segments. To archieve this, it connects one source-cell [z_in] to one destination-cell [z_out], and prompts a flow of cars with the rate Rk (Parameter) if and only if there are still cars at the end of [z_out] avaiable and if the capacity of [z_out] is not yet surpassed, i.e. (z_in x0 > 0 AND z_out Kz > z_out x), otherwise the flow is reduced to 0.
      settings: PortSchema="{\"entries\":[{\"content\":{\"sides\":[{\"content\":{\"connectorIds\":[\"In1\",\"Out2\",\"Out3\"]},\"type\":\"ConnectorPlacement.EquallySpacedRectSide\",\"uuid\":\"f9c1cf46-46ac-4011-8499-7a2e74fc4a3a\"},{\"content\":{\"connectorIds\":[\"In2\",\"In3\",\"Out1\"],\"side\":\"RIGHT\"},\"type\":\"ConnectorPlacement.EquallySpacedRectSide\",\"uuid\":\"f685a77a-a8b9-4a29-8679-dc3cbf3c2b7f\"},{\"content\":{\"connectorIds\":[],\"side\":\"TOP\"},\"type\":\"ConnectorPlacement.EquallySpacedRectSide\",\"uuid\":\"af8d715a-ddb3-4f5e-8163-596be4e65ef7\"}]},\"type\":\"ConnectorPlacement.EquallySpacedConnector\",\"uuid\":\"ace495d2-b7cd-4153-a555-4989f077c969\"}],\"packageUris\":[\"http://schema.mathworks.com/mf0/Connector/R2020b\"],\"version\":\"1.0\"}"
      mask Display:
      | image('$imagefile'); % Use "Edit Image" on toolstrip to change.
      | % image('$imagefile');
      | disp('Simple Edge 1x1 \n\n');
      | disp(['Rk = ', get_param(gcb,'Rk')])
  yk (dest) : Outport
  yk (source1) : Outport  Port=2
  yk (source2) : Outport  Port=3
  free_capacity_1 : Outport  Port=4
  free_capacity_2 : Outport  Port=5
  wires:
  z_out Kz/1 -> b/3(z_out Kz), a/3(z_out Kz)
  Sum/1 -> yk (dest)/1
  z_out x/1 -> b/2(z_out x), a/2(z_out x)
  b/1(yk (dest)) -> Sum/2
  z_in1 x0/1 -> a/1(z_in x0)
  a/1(yk (dest)) -> Sum/1
  z_in2 x0/1 -> b/1(z_in x0)
  b/2(yk (source)) -> yk (source2)/1
  a/2(yk (source)) -> yk (source1)/1
  a/3(free_capacity) -> free_capacity_1/1
  b/3(free_capacity) -> free_capacity_2/1

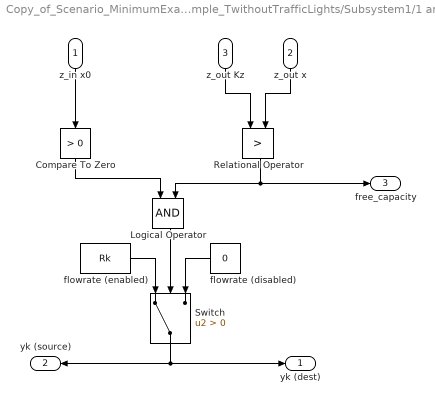
== system Copy_of_Scenario_MinimumExample_TwithoutTrafficLights/Subsystem1/1 and 2/a ==
  z_in x0 : Inport
  z_out x : Inport  Port=2
  z_out Kz : Inport  Port=3
  Compare To Zero : simulink/Logic and Bit Operations/Compare To Zero  relop=>  OutDataTypeStr=boolean
  Logical Operator : Logic  AllPortsSameDT=off  OutDataTypeStr=boolean
  Relational Operator : RelationalOperator  Operator=>  OutDataTypeStr=boolean  RndMeth=Simplest
  Switch : Switch  Criteria=u2 > Threshold
  flowrate (disabled) : Constant  Value=0
  flowrate (enabled) : Constant  Value=Rk
  yk (dest) : Outport
  yk (source) : Outport  Port=2
  free_capacity : Outport  Port=3
  wires:
  flowrate (disabled)/1 -> Switch/3
  z_in x0/1 -> Compare To Zero/1
  flowrate (enabled)/1 -> Switch/1
  Switch/1 -> yk (dest)/1, yk (source)/1
  z_out Kz/1 -> Relational Operator/1
  Logical Operator/1 -> Switch/2
  z_out x/1 -> Relational Operator/2
  Compare To Zero/1 -> Logical Operator/1
  Relational Operator/1 -> free_capacity/1, Logical Operator/2

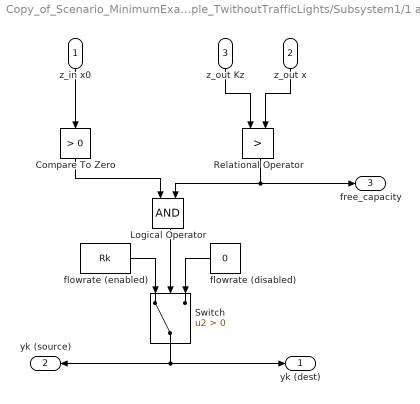
== system Copy_of_Scenario_MinimumExample_TwithoutTrafficLights/Subsystem1/1 and 2/b ==
  z_in x0 : Inport
  z_out x : Inport  Port=2
  z_out Kz : Inport  Port=3
  Compare To Zero : simulink/Logic and Bit Operations/Compare To Zero  relop=>  OutDataTypeStr=boolean
  Logical Operator : Logic  AllPortsSameDT=off  OutDataTypeStr=boolean
  Relational Operator : RelationalOperator  Operator=>  OutDataTypeStr=boolean  RndMeth=Simplest
  Switch : Switch  Criteria=u2 > Threshold
  flowrate (disabled) : Constant  Value=0
  flowrate (enabled) : Constant  Value=Rk
  yk (dest) : Outport
  yk (source) : Outport  Port=2
  free_capacity : Outport  Port=3
  wires:
  flowrate (disabled)/1 -> Switch/3
  z_in x0/1 -> Compare To Zero/1
  flowrate (enabled)/1 -> Switch/1
  Switch/1 -> yk (dest)/1, yk (source)/1
  z_out Kz/1 -> Relational Operator/1
  Logical Operator/1 -> Switch/2
  z_out x/1 -> Relational Operator/2
  Compare To Zero/1 -> Logical Operator/1
  Relational Operator/1 -> free_capacity/1, Logical Operator/2

== system Copy_of_Scenario_MinimumExample_TwithoutTrafficLights/Subsystem1/5 (bottom) and 6 (top)/a ==
  z_in x0 : Inport
  z_out x : Inport  Port=2
  z_out Kz : Inport  Port=3
  Compare To Zero : simulink/Logic and Bit Operations/Compare To Zero  relop=>  OutDataTypeStr=boolean
  Logical Operator : Logic  AllPortsSameDT=off  OutDataTypeStr=boolean
  Relational Operator : RelationalOperator  Operator=>  OutDataTypeStr=boolean  RndMeth=Simplest
  Switch : Switch  Criteria=u2 > Threshold
  flowrate (disabled) : Constant  Value=0
  flowrate (enabled) : Constant  Value=Rk
  yk (dest) : Outport
  yk (source) : Outport  Port=2
  free_capacity : Outport  Port=3
  wires:
  flowrate (disabled)/1 -> Switch/3
  z_in x0/1 -> Compare To Zero/1
  flowrate (enabled)/1 -> Switch/1
  Switch/1 -> yk (dest)/1, yk (source)/1
  z_out Kz/1 -> Relational Operator/1
  Logical Operator/1 -> Switch/2
  z_out x/1 -> Relational Operator/2
  Compare To Zero/1 -> Logical Operator/1
  Relational Operator/1 -> Logical Operator/2, free_capacity/1

== system Copy_of_Scenario_MinimumExample_TwithoutTrafficLights/Subsystem1/5 (bottom) and 6 (top)/b ==
  z_in x0 : Inport
  z_out x : Inport  Port=2
  z_out Kz : Inport  Port=3
  Compare To Zero : simulink/Logic and Bit Operations/Compare To Zero  relop=>  OutDataTypeStr=boolean
  Logical Operator : Logic  AllPortsSameDT=off  OutDataTypeStr=boolean
  Relational Operator : RelationalOperator  Operator=>  OutDataTypeStr=boolean  RndMeth=Simplest
  Switch : Switch  Criteria=u2 > Threshold
  flowrate (disabled) : Constant  Value=0
  flowrate (enabled) : Constant  Value=Rk
  yk (dest) : Outport
  yk (source) : Outport  Port=2
  free_capacity : Outport  Port=3
  wires:
  flowrate (disabled)/1 -> Switch/3
  z_in x0/1 -> Compare To Zero/1
  flowrate (enabled)/1 -> Switch/1
  Switch/1 -> yk (dest)/1, yk (source)/1
  z_out Kz/1 -> Relational Operator/1
  Logical Operator/1 -> Switch/2
  z_out x/1 -> Relational Operator/2
  Compare To Zero/1 -> Logical Operator/1
  Relational Operator/1 -> free_capacity/1, Logical Operator/2

== system Copy_of_Scenario_MinimumExample_TwithoutTrafficLights/Subsystem1/9 (top) and 10 (bottoM)/a ==
  z_in x0 : Inport
  z_out x : Inport  Port=2
  z_out Kz : Inport  Port=3
  Compare To Zero : simulink/Logic and Bit Operations/Compare To Zero  relop=>  OutDataTypeStr=boolean
  Logical Operator : Logic  AllPortsSameDT=off  OutDataTypeStr=boolean
  Relational Operator : RelationalOperator  Operator=>  OutDataTypeStr=boolean  RndMeth=Simplest
  Switch : Switch  Criteria=u2 > Threshold
  flowrate (disabled) : Constant  Value=0
  flowrate (enabled) : Constant  Value=Rk
  yk (dest) : Outport
  yk (source) : Outport  Port=2
  free_capacity : Outport  Port=3
  wires:
  flowrate (disabled)/1 -> Switch/3
  z_in x0/1 -> Compare To Zero/1
  flowrate (enabled)/1 -> Switch/1
  Switch/1 -> yk (dest)/1, yk (source)/1
  z_out Kz/1 -> Relational Operator/1
  Logical Operator/1 -> Switch/2
  z_out x/1 -> Relational Operator/2
  Compare To Zero/1 -> Logical Operator/1
  Relational Operator/1 -> free_capacity/1, Logical Operator/2

== system Copy_of_Scenario_MinimumExample_TwithoutTrafficLights/Subsystem1/9 (top) and 10 (bottoM)/b ==
  z_in x0 : Inport
  z_out x : Inport  Port=2
  z_out Kz : Inport  Port=3
  Compare To Zero : simulink/Logic and Bit Operations/Compare To Zero  relop=>  OutDataTypeStr=boolean
  Logical Operator : Logic  AllPortsSameDT=off  OutDataTypeStr=boolean
  Relational Operator : RelationalOperator  Operator=>  OutDataTypeStr=boolean  RndMeth=Simplest
  Switch : Switch  Criteria=u2 > Threshold
  flowrate (disabled) : Constant  Value=0
  flowrate (enabled) : Constant  Value=Rk
  yk (dest) : Outport
  yk (source) : Outport  Port=2
  free_capacity : Outport  Port=3
  wires:
  flowrate (disabled)/1 -> Switch/3
  z_in x0/1 -> Compare To Zero/1
  flowrate (enabled)/1 -> Switch/1
  Switch/1 -> yk (dest)/1, yk (source)/1
  z_out Kz/1 -> Relational Operator/1
  Logical Operator/1 -> Switch/2
  z_out x/1 -> Relational Operator/2
  Compare To Zero/1 -> Logical Operator/1
  Relational Operator/1 -> free_capacity/1, Logical Operator/2

== system Copy_of_Scenario_MinimumExample_TwithoutTrafficLights/Subsystem3/1 and 2/a ==
  z_in x0 : Inport
  z_out x : Inport  Port=2
  z_out Kz : Inport  Port=3
  Compare To Zero : simulink/Logic and Bit Operations/Compare To Zero  relop=>  OutDataTypeStr=boolean
  Logical Operator : Logic  AllPortsSameDT=off  OutDataTypeStr=boolean
  Relational Operator : RelationalOperator  Operator=>  OutDataTypeStr=boolean  RndMeth=Simplest
  Switch : Switch  Criteria=u2 > Threshold
  flowrate (disabled) : Constant  Value=0
  flowrate (enabled) : Constant  Value=Rk
  yk (dest) : Outport
  yk (source) : Outport  Port=2
  free_capacity : Outport  Port=3
  wires:
  flowrate (disabled)/1 -> Switch/3
  z_in x0/1 -> Compare To Zero/1
  flowrate (enabled)/1 -> Switch/1
  Switch/1 -> yk (dest)/1, yk (source)/1
  z_out Kz/1 -> Relational Operator/1
  Logical Operator/1 -> Switch/2
  z_out x/1 -> Relational Operator/2
  Compare To Zero/1 -> Logical Operator/1
  Relational Operator/1 -> free_capacity/1, Logical Operator/2

== system Copy_of_Scenario_MinimumExample_TwithoutTrafficLights/Subsystem3/1 and 2/b ==
  z_in x0 : Inport
  z_out x : Inport  Port=2
  z_out Kz : Inport  Port=3
  Compare To Zero : simulink/Logic and Bit Operations/Compare To Zero  relop=>  OutDataTypeStr=boolean
  Logical Operator : Logic  AllPortsSameDT=off  OutDataTypeStr=boolean
  Relational Operator : RelationalOperator  Operator=>  OutDataTypeStr=boolean  RndMeth=Simplest
  Switch : Switch  Criteria=u2 > Threshold
  flowrate (disabled) : Constant  Value=0
  flowrate (enabled) : Constant  Value=Rk
  yk (dest) : Outport
  yk (source) : Outport  Port=2
  free_capacity : Outport  Port=3
  wires:
  flowrate (disabled)/1 -> Switch/3
  z_in x0/1 -> Compare To Zero/1
  flowrate (enabled)/1 -> Switch/1
  Switch/1 -> yk (dest)/1, yk (source)/1
  z_out Kz/1 -> Relational Operator/1
  Logical Operator/1 -> Switch/2
  z_out x/1 -> Relational Operator/2
  Compare To Zero/1 -> Logical Operator/1
  Relational Operator/1 -> free_capacity/1, Logical Operator/2

== system Copy_of_Scenario_MinimumExample_TwithoutTrafficLights/Subsystem3/5 (bottom) and 6 (top)/a ==
  z_in x0 : Inport
  z_out x : Inport  Port=2
  z_out Kz : Inport  Port=3
  Compare To Zero : simulink/Logic and Bit Operations/Compare To Zero  relop=>  OutDataTypeStr=boolean
  Logical Operator : Logic  AllPortsSameDT=off  OutDataTypeStr=boolean
  Relational Operator : RelationalOperator  Operator=>  OutDataTypeStr=boolean  RndMeth=Simplest
  Switch : Switch  Criteria=u2 > Threshold
  flowrate (disabled) : Constant  Value=0
  flowrate (enabled) : Constant  Value=Rk
  yk (dest) : Outport
  yk (source) : Outport  Port=2
  free_capacity : Outport  Port=3
  wires:
  flowrate (disabled)/1 -> Switch/3
  z_in x0/1 -> Compare To Zero/1
  flowrate (enabled)/1 -> Switch/1
  Switch/1 -> yk (dest)/1, yk (source)/1
  z_out Kz/1 -> Relational Operator/1
  Logical Operator/1 -> Switch/2
  z_out x/1 -> Relational Operator/2
  Compare To Zero/1 -> Logical Operator/1
  Relational Operator/1 -> Logical Operator/2, free_capacity/1

== system Copy_of_Scenario_MinimumExample_TwithoutTrafficLights/Subsystem3/5 (bottom) and 6 (top)/b ==
  z_in x0 : Inport
  z_out x : Inport  Port=2
  z_out Kz : Inport  Port=3
  Compare To Zero : simulink/Logic and Bit Operations/Compare To Zero  relop=>  OutDataTypeStr=boolean
  Logical Operator : Logic  AllPortsSameDT=off  OutDataTypeStr=boolean
  Relational Operator : RelationalOperator  Operator=>  OutDataTypeStr=boolean  RndMeth=Simplest
  Switch : Switch  Criteria=u2 > Threshold
  flowrate (disabled) : Constant  Value=0
  flowrate (enabled) : Constant  Value=Rk
  yk (dest) : Outport
  yk (source) : Outport  Port=2
  free_capacity : Outport  Port=3
  wires:
  flowrate (disabled)/1 -> Switch/3
  z_in x0/1 -> Compare To Zero/1
  flowrate (enabled)/1 -> Switch/1
  Switch/1 -> yk (dest)/1, yk (source)/1
  z_out Kz/1 -> Relational Operator/1
  Logical Operator/1 -> Switch/2
  z_out x/1 -> Relational Operator/2
  Compare To Zero/1 -> Logical Operator/1
  Relational Operator/1 -> free_capacity/1, Logical Operator/2

== system Copy_of_Scenario_MinimumExample_TwithoutTrafficLights/Subsystem3/9 (top) and 10 (bottoM)/a ==
  z_in x0 : Inport
  z_out x : Inport  Port=2
  z_out Kz : Inport  Port=3
  Compare To Zero : simulink/Logic and Bit Operations/Compare To Zero  relop=>  OutDataTypeStr=boolean
  Logical Operator : Logic  AllPortsSameDT=off  OutDataTypeStr=boolean
  Relational Operator : RelationalOperator  Operator=>  OutDataTypeStr=boolean  RndMeth=Simplest
  Switch : Switch  Criteria=u2 > Threshold
  flowrate (disabled) : Constant  Value=0
  flowrate (enabled) : Constant  Value=Rk
  yk (dest) : Outport
  yk (source) : Outport  Port=2
  free_capacity : Outport  Port=3
  wires:
  flowrate (disabled)/1 -> Switch/3
  z_in x0/1 -> Compare To Zero/1
  flowrate (enabled)/1 -> Switch/1
  Switch/1 -> yk (dest)/1, yk (source)/1
  z_out Kz/1 -> Relational Operator/1
  Logical Operator/1 -> Switch/2
  z_out x/1 -> Relational Operator/2
  Compare To Zero/1 -> Logical Operator/1
  Relational Operator/1 -> free_capacity/1, Logical Operator/2

== system Copy_of_Scenario_MinimumExample_TwithoutTrafficLights/Subsystem3/9 (top) and 10 (bottoM)/b ==
  z_in x0 : Inport
  z_out x : Inport  Port=2
  z_out Kz : Inport  Port=3
  Compare To Zero : simulink/Logic and Bit Operations/Compare To Zero  relop=>  OutDataTypeStr=boolean
  Logical Operator : Logic  AllPortsSameDT=off  OutDataTypeStr=boolean
  Relational Operator : RelationalOperator  Operator=>  OutDataTypeStr=boolean  RndMeth=Simplest
  Switch : Switch  Criteria=u2 > Threshold
  flowrate (disabled) : Constant  Value=0
  flowrate (enabled) : Constant  Value=Rk
  yk (dest) : Outport
  yk (source) : Outport  Port=2
  free_capacity : Outport  Port=3
  wires:
  flowrate (disabled)/1 -> Switch/3
  z_in x0/1 -> Compare To Zero/1
  flowrate (enabled)/1 -> Switch/1
  Switch/1 -> yk (dest)/1, yk (source)/1
  z_out Kz/1 -> Relational Operator/1
  Logical Operator/1 -> Switch/2
  z_out x/1 -> Relational Operator/2
  Compare To Zero/1 -> Logical Operator/1
  Relational Operator/1 -> free_capacity/1, Logical Operator/2

== stateflow chart Copy_of_Scenario_MinimumExample_TwithoutTrafficLights/Plus-Controller ==
  note: ?
  state Group__Crs_Brs
  state Group__Cl_Bl
  state Group__Ars_Drs
  state Group__Al_Dl
  note: check
      | Crs straight
      | crossings
  note: check
      | Cl
      | crossings
  note: check
      | Ars straight
      | crossings
  note: check
      | Al
      | crossings
  note: check
      | Crs right
      | crossings
  note: check
      | Bl
      | crossings
  note: check
      | Ars right
      | crossings
  note: check
      | Dl
      | crossings
  note: check
      | Brs straight
      | crossings
  note: check
      | Drs straight
      | crossings
  note: check
      | Brs right
      | crossings
  note: check
      | Drs right
      | crossings
  Group__Al_Dl -> Group__Crs_Brs [order 2] : [[[after(green_duration_l, sec)]]]
      | {enAl = 0; enDl = 0;}
  Group__Ars_Drs -> Group__Al_Dl [order 1] : [[after(green_duration_sr, sec)]]
      | {enAs = 0; enAr = 0; enDs = 0; enDr = 0;}
  Group__Cl_Bl -> Group__Ars_Drs [order 1] : [after(green_duration_l, sec)]
      | {enCl = 0; enBl = 0;}
  Group__Crs_Brs -> Group__Cl_Bl [order 1] : [after(green_duration_sr, sec)]
      | {enCs = 0; enCr = 0; ...
      | enBs = 0; enBr = 0;}
  (default) -> Group__Crs_Brs : {enAl = 0; enAs = 0; enAr = 0;
      | enBl = 0; enBs = 0; enBr = 0;
      | enCl = 0; enCs = 0; enCr = 0;
      | enDl = 0; enDs = 0; enDr = 0;}
  Group__Crs_Brs -> (junction 51) [order 2]
  (junction 109) -> Group__Crs_Brs
  Group__Cl_Bl -> (junction 117) [order 2]
  (junction 126) -> Group__Cl_Bl
  Group__Ars_Drs -> (junction 134) [order 2]
  (junction 131) -> Group__Ars_Drs
  Group__Al_Dl -> (junction 151) [order 1]
  (junction 160) -> Group__Al_Dl
  (junction 117) -> (junction 116) [order 2] : {enCl = 0;}
  (junction 51) -> (junction 59) [order 1] : [(Dl_Co==0 && Drs_Ao==0 ...
      | && Drs_Bo==0 && Bl_Do==0 ...
      | && Al_Bo==0 && Ars_Do==0)]
      | {enCs = 1;}
  (junction 117) -> (junction 116) [order 1] : [(Dl_Co==0 && Drs_Ao==0 && ....
      | Brs_Co==0 && Al_Bo==0 && ...
      | Ars_Do==0)]{enCl = 1;}
  (junction 51) -> (junction 59) [order 2] : {enCs = 0;}
  (junction 134) -> (junction 133) [order 1] : [((Cl_Ao==0 && Crs_Bo==0 && ...
      | Crs_Do==0 && Dl_Co==0 && ...
      | Bl_Do==0 && Brs_Co==0))]
      | {enAs = 1;}
  (junction 151) -> (junction 150) [order 1] : [(Cl_Ao==0 && Crs_Bo==0 ...
      | && Drs_Ao==0 && Bl_Do==0 ...
      | && Brs_Co==0)]{enAl = 1;}
  (junction 134) -> (junction 133) [order 2] : {enAs = 0;}
  (junction 151) -> (junction 150) [order 2] : {enAl = 0;}
  (junction 59) -> (junction 104) [order 1] : [(Ars_Do==0 && Bl_Do==0)]
      | {enCr = 1;}
  (junction 116) -> (junction 126) [order 1] : [(Al_Bo==0 && Ars_Do==0 && ...
      | Crs_Bo==0 && Dl_Co==0 && ...
      | Drs_Ao==0)]{enBl = 1;}
  (junction 59) -> (junction 104) [order 2] : {enCr = 0;}
  (junction 116) -> (junction 126) [order 2] : {enBl = 0;}
  (junction 133) -> (junction 143) [order 1] : [(Brs_Co==0 && Dl_Co==0)]
      | {enAr = 1;}
  (junction 150) -> (junction 160) [order 1] : [(Bl_Do==0 && Brs_Co==0 ...
      | && Ars_Do==0 && Cl_Ao==0 ...
      | && Crs_Bo==0)]{enDl = 1;}
  (junction 133) -> (junction 143) [order 2] : {enAr = 0;}
  (junction 150) -> (junction 160) [order 2] : {enDl = 0;}
  (junction 104) -> (junction 105) [order 1] : [(Al_Bo==0 && Ars_Do==0 ...
      | && Ars_Co==0 && Cl_Ao==0 ...
      | && Dl_Co==0 && Drs_Ao==0)]
      | {enBs = 1;}
  (junction 104) -> (junction 105) [order 2] : {enBs = 0;}
  (junction 143) -> (junction 141) [order 1] : [(Bl_Do==0 && Brs_Co==0 ...
      | && Brs_Ao==0 && Al_Bo==0 ...
      | && Cl_Ao==0 && Crs_Bo==0)]
      | {enDs = 1;}
  (junction 143) -> (junction 141) [order 2] : {enDs=0;}
  (junction 105) -> (junction 109) [order 1] : [Drs_Ao==0 && Cl_Ao==0]
      | {enBr = 1;}
  (junction 105) -> (junction 109) [order 2] : {enBr = 0;}
  (junction 141) -> (junction 131) [order 1] : [(Crs_Bo==0 && Al_Bo==0)]
      | {enDr = 1;}
  (junction 141) -> (junction 131) [order 2] : {enDr = 0;}
  data: Bl input; Brs input; Al input; Ars input; Cl input; Crs input; Dl input; Drs input; Al_Bo input; Ars_Do input; Ars_Co input; Bl_Do input; Brs_Co input; Brs_Ao input; Cl_Ao input; Crs_Bo input; Crs_Do input; Dl_Co input; Drs_Ao input; Drs_Bo input; enAl output =0; enAs output =0; enAr output =0; enBl output =0; enBs output =0; enBr output =0; enCl output =0; enCs output =0; enCr output =0; enDl output =0; enDs output =0; enDr output =0; green_duration_sr parameter; green_duration_l parameter
